simulink model "homework2_cont"  (R2019a)
settings: Solver=VariableStepAuto  StartTime=0.0  StopTime=10  RelTol=1e-3
values from neighbouring files (symbols this model uses):
  b = 100    [homework2.m]
  K_i = 638    [homework2.m]
  K_p = 1050    [homework2.m]
  m = 1000    [homework2.m]
settings Model: Creator=lucanhen  LastModifiedBy=lucanhen

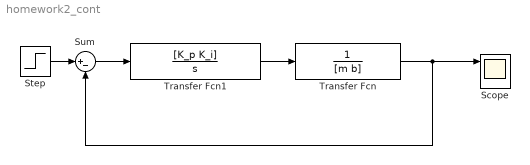
== system homework2_cont ==
  Scope : Scope  NumInputPorts=3
  Step : Step  Time=0  After=100  SampleTime=0
  Sum : Sum  Inputs=|+-
  Transfer Fcn : TransferFcn  Denominator=[m b]
  Transfer Fcn1 : TransferFcn  Numerator=[K_p K_i]  Denominator=[1 0]
  wires:
  Step/1 -> Sum/1
  Transfer Fcn/1 -> Sum/2, Scope/1
  Transfer Fcn1/1 -> Transfer Fcn/1
  Sum/1 -> Transfer Fcn1/1
